simulink model "DAC_fxn_neg"  (R2018b)
settings: Solver=VariableStepAuto  StartTime=0.0  StopTime=10.0  RelTol=1e-3
libraries: simulink_extras x36, simulink x1
settings Model: Creator=iamcy  LastModifiedBy=iamcy

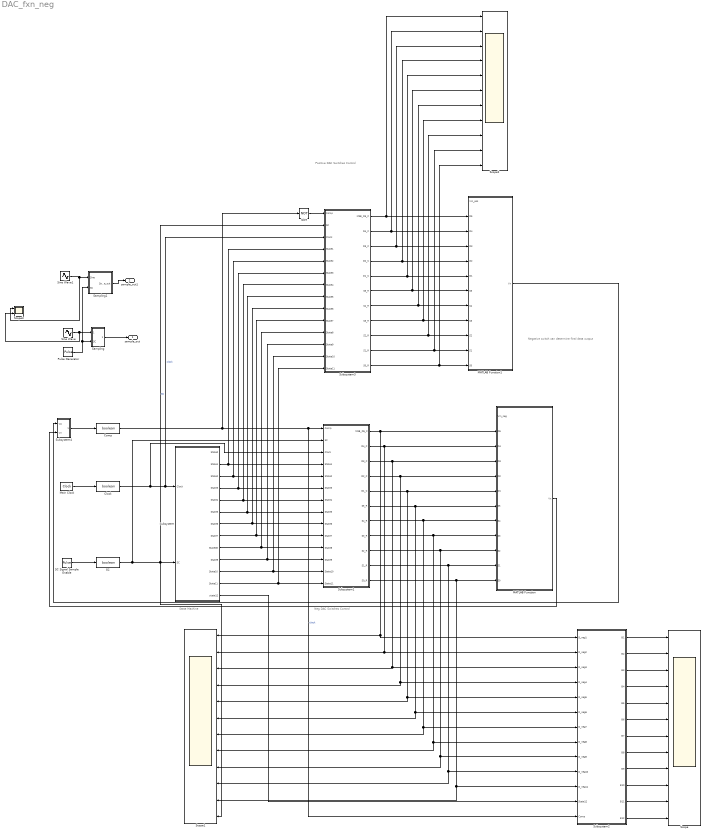
== system DAC_fxn_neg ==
  note: Negative switch can determine final data output
  note: Neg DAC Switches Control
  note: State Machine
  note: Positive DAC Switches Control
  Clock : DataTypeConversion  OutDataTypeStr=boolean
  Comp : DataTypeConversion  OutDataTypeStr=boolean
  MATLAB Function : MATLAB Function  TreatAsAtomicUnit=on
  MATLAB Function1 : MATLAB Function  TreatAsAtomicUnit=on
  Main Clock : simulink_extras/Flip Flops/Clock  period=1
  NOT : Logic  Operator=NOT  IconShape=distinctive  AllPortsSameDT=off  OutDataTypeStr=boolean
  Pulse Generator : DiscretePulseGenerator  PulseType=Time based  Period=13  PulseWidth=100/13
  SC : DataTypeConversion  OutDataTypeStr=boolean
  SC Signal Sample Enable : DiscretePulseGenerator  PulseType=Time based  Period=13  PulseWidth=100/13
  Sampling : Subsystem
  Sampling1 : Subsystem
  Scope : Scope  NumInputPorts=12
  Scope1 : Scope  NumInputPorts=12
  Scope2 : Scope  NumInputPorts=11
  Scope3 : Scope  NumInputPorts=2
  Sine Wave : Sin  Frequency=0.01  Phase=pi  SampleTime=0
  Sine Wave1 : Sin  Frequency=0.01  SampleTime=0
  Subsystem : Subsystem
  Subsystem1 : Subsystem
  Subsystem2 : Subsystem
  Subsystem3 : Subsystem
  Subsystem4 : Subsystem
  sample_out : Outport
  sample_out1 : Outport  Port=2
  wires:
  Subsystem/13(state12) -> Subsystem2/12(State12)
  Subsystem1/9(S2_R) -> MATLAB Function/10(S2), Scope1/9, Subsystem2/9(D_neg9)
  Subsystem1/11(S0_R) -> MATLAB Function/12(S0), Scope1/11, Subsystem2/11(D_neg11)
  Subsystem1/8(S3_R) -> MATLAB Function/9(S3), Scope1/8, Subsystem2/8(D_neg8)
  Subsystem1/6(S5_R) -> MATLAB Function/7(S5), Scope1/6, Subsystem2/6(D_neg6)
  Subsystem1/5(D1_C) -> MATLAB Function/6(D1), Scope1/5, Subsystem2/5(D_neg5)
  Subsystem1/3(D3_C) -> MATLAB Function/4(D3), Scope1/3, Subsystem2/3(D_neg3)
  Subsystem1/2(D4_C) -> MATLAB Function/3(D4), Scope1/2, Subsystem2/2(D_neg2)
  Subsystem1/1(MSB_D5_C) -> MATLAB Function/2(D5), Scope1/1, Subsystem2/1(D_neg1)
  Subsystem4/1(Comp) -> Comp/1
  Subsystem1/4(D2_C) -> MATLAB Function/5(D2), Scope1/4, Subsystem2/4(D_neg4)
  Comp/1 -> NOT/1, Subsystem2/13(Comp), Subsystem1/1(Comp)  "clock"
  Subsystem2/9(B9) -> Scope/9
  Subsystem2/12(B12) -> Scope/12
  Subsystem2/10(B10) -> Scope/10
  Subsystem2/7(B7) -> Scope/7
  Subsystem2/6(B6) -> Scope/6
  Subsystem2/3(B3) -> Scope/3
  Subsystem2/5(B5) -> Scope/5
  Subsystem2/2(B2) -> Scope/2
  Subsystem2/1(B1) -> Scope/1
  SC Signal Sample Enable/1 -> SC/1
  Main Clock/1 -> Clock/1
  Clock/1 -> Subsystem1/3(Clock), Subsystem3/3(Clock), Subsystem/1(Clock)  "clock"
  Subsystem2/4(B4) -> Scope/4
  Subsystem3/7(S4_R) -> MATLAB Function1/8(S4), Scope2/7
  Subsystem3/5(D1_C) -> MATLAB Function1/6(D1), Scope2/5
  Subsystem1/7(S4_R) -> MATLAB Function/8(S4), Scope1/7, Subsystem2/7(D_neg7)
  Subsystem3/9(S2_R) -> MATLAB Function1/10(S2), Scope2/9
  Subsystem2/11(B11) -> Scope/11
  Subsystem1/10(S1_R) -> MATLAB Function/11(S1), Scope1/10, Subsystem2/10(D_neg10)
  Subsystem3/3(D3_C) -> MATLAB Function1/4(D3), Scope2/3
  Subsystem3/1(MSB_D5_C) -> MATLAB Function1/2(D5), Scope2/1
  Subsystem2/8(B8) -> Scope/8
  NOT/1 -> Subsystem3/1(Comp)
  Subsystem3/8(S3_R) -> MATLAB Function1/9(S3), Scope2/8
  Subsystem3/6(S5_R) -> MATLAB Function1/7(S5), Scope2/6
  Subsystem3/10(S1_R) -> MATLAB Function1/11(S1), Scope2/10
  Subsystem3/2(D4_C) -> MATLAB Function1/3(D4), Scope2/2
  Subsystem3/4(D2_C) -> MATLAB Function1/5(D2), Scope2/4
  Subsystem3/11(S0_R) -> MATLAB Function1/12(S0), Scope2/11
  Subsystem/11(State10) -> Subsystem3/13(State10), Subsystem1/13(State10)
  Subsystem/9(State08) -> Subsystem3/11(State8), Subsystem1/11(State8)
  Subsystem/10(State9) -> Subsystem3/12(State9), Subsystem1/12(State9)
  Subsystem/7(State6) -> Subsystem3/9(State6), Subsystem1/9(State6)
  Subsystem/12(State11) -> Subsystem3/14(State11), Subsystem1/14(State11)
  Subsystem/8(State7) -> Subsystem3/10(State7), Subsystem1/10(State7)
  Subsystem/4(State3) -> Subsystem3/6(State3), Subsystem1/6(State3)
  Subsystem/5(State4) -> Subsystem3/7(State4), Subsystem1/7(State4)
  SC/1 -> Subsystem1/2(SC), Scope1/12, Subsystem3/2(SC), Subsystem/2(SC)  "SC"
  Subsystem/3(State2) -> Subsystem3/5(State2), Subsystem1/5(State2)
  Subsystem/6(State5) -> Subsystem3/8(State5), Subsystem1/8(State5)
  Subsystem/2(State1) -> Subsystem3/4(State1), Subsystem1/4(State1)
  MATLAB Function1/1(Vx) -> Subsystem4/1(Vp)
  MATLAB Function/1(Vx) -> Subsystem4/2(Vn)
  Sampling/1(Sample_out) -> sample_out/1
  Sine Wave/1 -> Scope3/2, Sampling/1(Sine)
  Pulse Generator/1 -> Sampling1/2(SC), Sampling/2(SC)
  Sampling1/1(Sample_out) -> sample_out1/1
  Sine Wave1/1 -> Scope3/1, Sampling1/1(Sine)

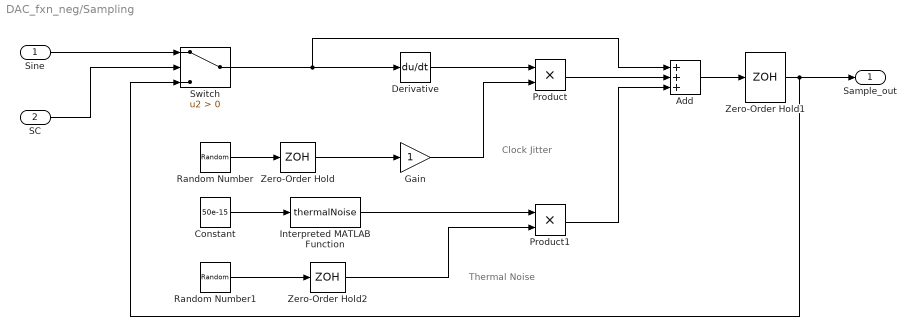
== system DAC_fxn_neg/Sampling ==
  note: Clock Jitter
  note: Thermal Noise
  Sine : Inport
  SC : Inport  Port=2
  Add : Sum  Inputs=3
  Constant : Constant  Value=50e-15
  Derivative : Derivative  CoefficientInTFapproximation=0
  Gain : Gain
  Interpreted MATLAB Function : MATLABFcn  MATLABFcn=thermalNoise
  Product : Product
  Product1 : Product
  Random Number : RandomNumber  Variance=30e-12  SampleTime=0.1
  Random Number1 : RandomNumber  Variance=30e-12  SampleTime=0.1
  Switch : Switch  Criteria=u2 > Threshold
  Zero-Order Hold : ZeroOrderHold  SampleTime=-1
  Zero-Order Hold1 : ZeroOrderHold  SampleTime=13
  Zero-Order Hold2 : ZeroOrderHold  SampleTime=-1
  Sample_out : Outport
  wires:
  Random Number/1 -> Zero-Order Hold/1
  Random Number1/1 -> Zero-Order Hold2/1
  Zero-Order Hold2/1 -> Product1/2
  Derivative/1 -> Product/1
  Interpreted MATLAB Function/1 -> Product1/1
  Product/1 -> Add/2
  Constant/1 -> Interpreted MATLAB Function/1
  Zero-Order Hold1/1 -> Sample_out/1, Switch/3
  Switch/1 -> Add/1, Derivative/1
  Zero-Order Hold/1 -> Gain/1
  Add/1 -> Zero-Order Hold1/1
  Gain/1 -> Product/2
  Product1/1 -> Add/3
  SC/1 -> Switch/2
  Sine/1 -> Switch/1

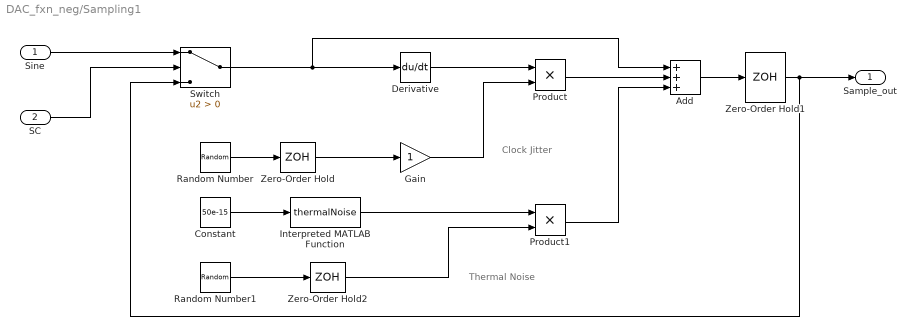
== system DAC_fxn_neg/Sampling1 ==
  note: Clock Jitter
  note: Thermal Noise
  Sine : Inport
  SC : Inport  Port=2
  Add : Sum  Inputs=3
  Constant : Constant  Value=50e-15
  Derivative : Derivative  CoefficientInTFapproximation=0
  Gain : Gain
  Interpreted MATLAB Function : MATLABFcn  MATLABFcn=thermalNoise
  Product : Product
  Product1 : Product
  Random Number : RandomNumber  Variance=30e-12  SampleTime=0.1
  Random Number1 : RandomNumber  Variance=30e-12  SampleTime=0.1
  Switch : Switch  Criteria=u2 > Threshold
  Zero-Order Hold : ZeroOrderHold  SampleTime=-1
  Zero-Order Hold1 : ZeroOrderHold  SampleTime=13
  Zero-Order Hold2 : ZeroOrderHold  SampleTime=-1
  Sample_out : Outport
  wires:
  Random Number/1 -> Zero-Order Hold/1
  Random Number1/1 -> Zero-Order Hold2/1
  Zero-Order Hold2/1 -> Product1/2
  Derivative/1 -> Product/1
  Interpreted MATLAB Function/1 -> Product1/1
  Product/1 -> Add/2
  Constant/1 -> Interpreted MATLAB Function/1
  Zero-Order Hold1/1 -> Sample_out/1, Switch/3
  Switch/1 -> Add/1, Derivative/1
  Zero-Order Hold/1 -> Gain/1
  Add/1 -> Zero-Order Hold1/1
  Gain/1 -> Product/2
  Product1/1 -> Add/3
  SC/1 -> Switch/2
  Sine/1 -> Switch/1

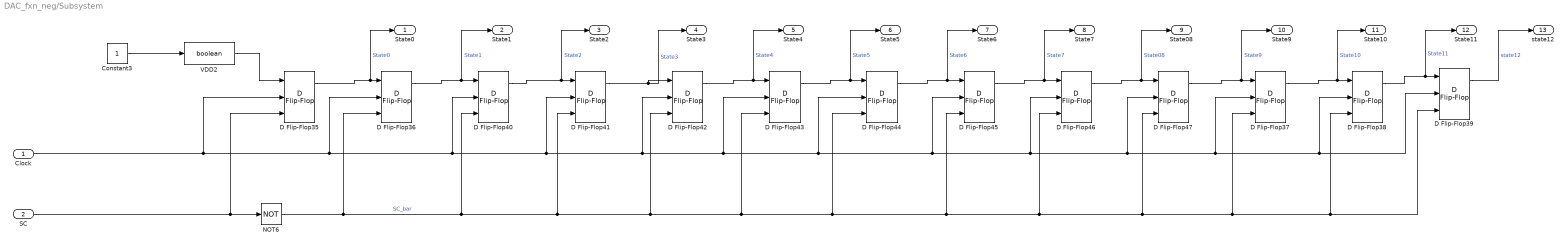
== system DAC_fxn_neg/Subsystem ==
  Clock : Inport
  SC : Inport  Port=2
  Constant3 : Constant
  D Flip-Flop{35..47} (13 alike) : simulink_extras/Flip Flops/D Flip-Flop
      settings: SourceProductName=Simulink
  NOT6 : Logic  Operator=NOT  IconShape=distinctive  AllPortsSameDT=off  OutDataTypeStr=boolean
  VDD2 : DataTypeConversion  OutDataTypeStr=boolean
  State0 : Outport
  State1 : Outport  Port=2
  State2 : Outport  Port=3
  State3 : Outport  Port=4
  State4 : Outport  Port=5
  State5 : Outport  Port=6
  State6 : Outport  Port=7
  State7 : Outport  Port=8
  State08 : Outport  Port=9
  State9 : Outport  Port=10
  State10 : Outport  Port=11
  State11 : Outport  Port=12
  state12 : Outport  Port=13
  wires:
  D Flip-Flop43/1 -> State5/1, D Flip-Flop44/1  "State5"
  D Flip-Flop40/1 -> State2/1, D Flip-Flop41/1  "State2"
  D Flip-Flop45/1 -> State7/1, D Flip-Flop46/1  "State7"
  D Flip-Flop38/1 -> State11/1, D Flip-Flop39/1  "State11"
  D Flip-Flop42/1 -> State4/1, D Flip-Flop43/1  "State4"
  D Flip-Flop44/1 -> State6/1, D Flip-Flop45/1  "State6"
  NOT6/1 -> D Flip-Flop42/3, D Flip-Flop44/3, D Flip-Flop46/3, D Flip-Flop38/3, D Flip-Flop39/3, D Flip-Flop37/3, D Flip-Flop47/3, D Flip-Flop45/3, D Flip-Flop43/3, D Flip-Flop41/3, D Flip-Flop40/3, D Flip-Flop36/3  "SC_bar"
  D Flip-Flop36/1 -> State1/1, D Flip-Flop40/1  "State1"
  Clock/1 -> D Flip-Flop36/2, D Flip-Flop41/2, D Flip-Flop42/2, D Flip-Flop43/2, D Flip-Flop44/2, D Flip-Flop45/2, D Flip-Flop46/2, D Flip-Flop38/2, D Flip-Flop39/2, D Flip-Flop37/2, D Flip-Flop47/2, D Flip-Flop40/2, D Flip-Flop35/2
  D Flip-Flop47/1 -> State9/1, D Flip-Flop37/1  "State9"
  Constant3/1 -> VDD2/1
  D Flip-Flop41/1 -> State3/1, D Flip-Flop42/1  "State3"
  D Flip-Flop37/1 -> State10/1, D Flip-Flop38/1  "State10"
  D Flip-Flop35/1 -> State0/1, D Flip-Flop36/1  "State0"
  D Flip-Flop46/1 -> State08/1, D Flip-Flop47/1  "State08"
  SC/1 -> NOT6/1, D Flip-Flop35/3
  VDD2/1 -> D Flip-Flop35/1
  D Flip-Flop39/1 -> state12/1  "state12"

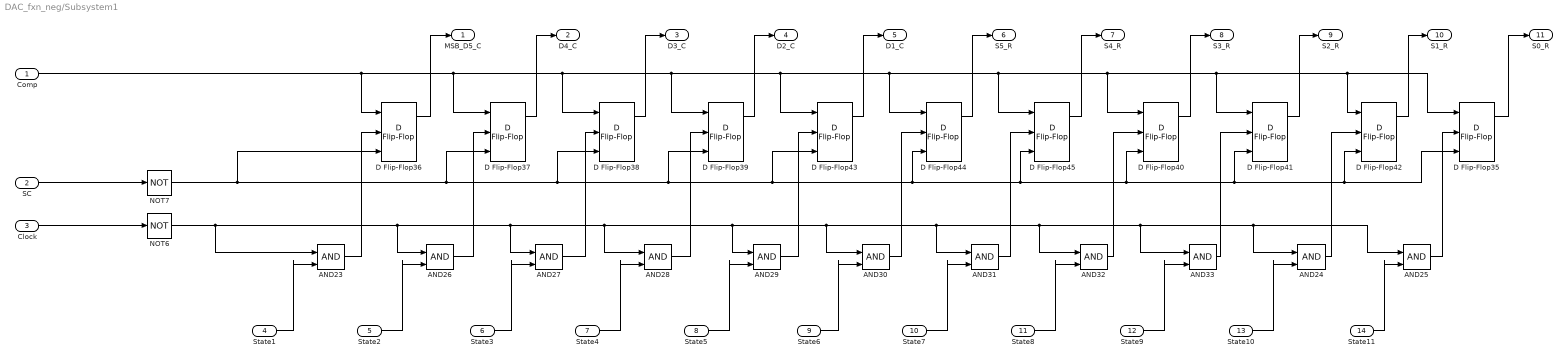
== system DAC_fxn_neg/Subsystem1 ==
  Comp : Inport
  SC : Inport  Port=2
  Clock : Inport  Port=3
  State1 : Inport  Port=4
  State2 : Inport  Port=5
  State3 : Inport  Port=6
  State4 : Inport  Port=7
  State5 : Inport  Port=8
  State6 : Inport  Port=9
  State7 : Inport  Port=10
  State8 : Inport  Port=11
  State9 : Inport  Port=12
  State10 : Inport  Port=13
  State11 : Inport  Port=14
  AND{23..33} (11 alike) : Logic  IconShape=distinctive  AllPortsSameDT=off  OutDataTypeStr=boolean
  D Flip-Flop{35..45} (11 alike) : simulink_extras/Flip Flops/D Flip-Flop
      settings: SourceProductName=Simulink
  NOT6 : Logic  Operator=NOT  IconShape=distinctive  AllPortsSameDT=off  OutDataTypeStr=boolean
  NOT7 : Logic  Operator=NOT  IconShape=distinctive  AllPortsSameDT=off  OutDataTypeStr=boolean
  MSB_D5_C : Outport
  D4_C : Outport  Port=2
  D3_C : Outport  Port=3
  D2_C : Outport  Port=4
  D1_C : Outport  Port=5
  S5_R : Outport  Port=6
  S4_R : Outport  Port=7
  S3_R : Outport  Port=8
  S2_R : Outport  Port=9
  S1_R : Outport  Port=10
  S0_R : Outport  Port=11
  wires:
  NOT7/1 -> D Flip-Flop35/3, D Flip-Flop42/3, D Flip-Flop41/3, D Flip-Flop40/3, D Flip-Flop45/3, D Flip-Flop44/3, D Flip-Flop43/3, D Flip-Flop39/3, D Flip-Flop38/3, D Flip-Flop37/3, D Flip-Flop36/3
  D Flip-Flop41/1 -> S2_R/1
  AND23/1 -> D Flip-Flop36/2
  State9/1 -> AND33/2
  Comp/1 -> D Flip-Flop35/1, D Flip-Flop42/1, D Flip-Flop41/1, D Flip-Flop40/1, D Flip-Flop45/1, D Flip-Flop44/1, D Flip-Flop43/1, D Flip-Flop39/1, D Flip-Flop38/1, D Flip-Flop37/1, D Flip-Flop36/1
  D Flip-Flop42/1 -> S1_R/1
  AND27/1 -> D Flip-Flop38/2
  NOT6/1 -> AND25/1, AND24/1, AND33/1, AND32/1, AND31/1, AND30/1, AND29/1, AND28/1, AND27/1, AND26/1, AND23/1
  AND25/1 -> D Flip-Flop35/2
  AND29/1 -> D Flip-Flop43/2
  AND31/1 -> D Flip-Flop45/2
  AND28/1 -> D Flip-Flop39/2
  State1/1 -> AND23/2
  AND33/1 -> D Flip-Flop41/2
  D Flip-Flop45/1 -> S4_R/1
  State5/1 -> AND29/2
  AND26/1 -> D Flip-Flop37/2
  AND24/1 -> D Flip-Flop42/2
  SC/1 -> NOT7/1
  AND32/1 -> D Flip-Flop40/2
  State10/1 -> AND24/2
  AND30/1 -> D Flip-Flop44/2
  D Flip-Flop38/1 -> D3_C/1
  Clock/1 -> NOT6/1
  D Flip-Flop36/1 -> MSB_D5_C/1
  D Flip-Flop37/1 -> D4_C/1
  D Flip-Flop35/1 -> S0_R/1
  D Flip-Flop43/1 -> D1_C/1
  State4/1 -> AND28/2
  State3/1 -> AND27/2
  State2/1 -> AND26/2
  State8/1 -> AND32/2
  D Flip-Flop44/1 -> S5_R/1
  State6/1 -> AND30/2
  State11/1 -> AND25/2
  D Flip-Flop40/1 -> S3_R/1
  State7/1 -> AND31/2
  D Flip-Flop39/1 -> D2_C/1

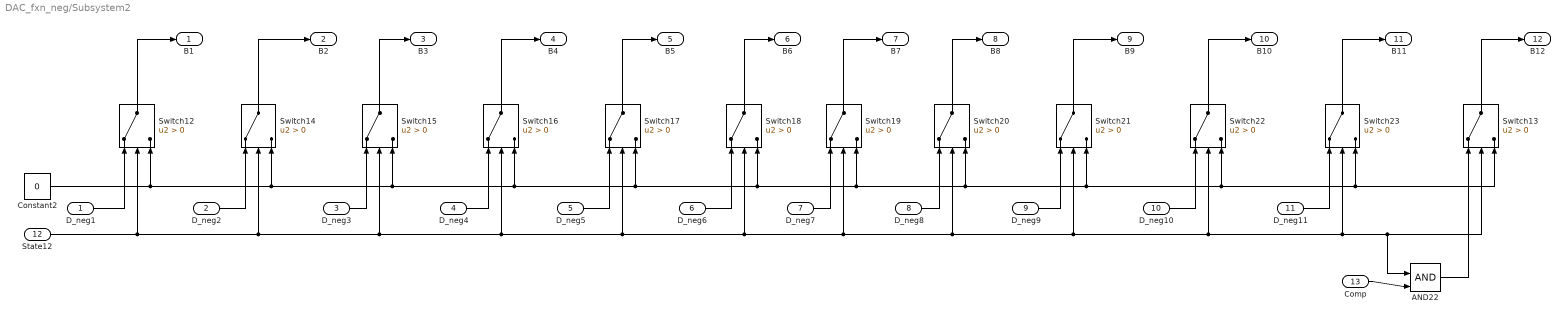
== system DAC_fxn_neg/Subsystem2 ==
  D_neg1 : Inport
  D_neg2 : Inport  Port=2
  D_neg3 : Inport  Port=3
  D_neg4 : Inport  Port=4
  D_neg5 : Inport  Port=5
  D_neg6 : Inport  Port=6
  D_neg7 : Inport  Port=7
  D_neg8 : Inport  Port=8
  D_neg9 : Inport  Port=9
  D_neg10 : Inport  Port=10
  D_neg11 : Inport  Port=11
  State12 : Inport  Port=12
  Comp : Inport  Port=13
  AND22 : Logic  IconShape=distinctive  AllPortsSameDT=off  OutDataTypeStr=boolean
  Constant2 : Constant  Value=0
  Switch{12..23} (12 alike) : Switch  Criteria=u2 > Threshold
  B1 : Outport
  B2 : Outport  Port=2
  B3 : Outport  Port=3
  B4 : Outport  Port=4
  B5 : Outport  Port=5
  B6 : Outport  Port=6
  B7 : Outport  Port=7
  B8 : Outport  Port=8
  B9 : Outport  Port=9
  B10 : Outport  Port=10
  B11 : Outport  Port=11
  B12 : Outport  Port=12
  wires:
  Constant2/1 -> Switch12/3, Switch13/3, Switch23/3, Switch22/3, Switch21/3, Switch20/3, Switch19/3, Switch18/3, Switch17/3, Switch16/3, Switch15/3, Switch14/3
  Switch22/1 -> B10/1
  Switch17/1 -> B5/1
  Switch12/1 -> B1/1
  Switch14/1 -> B2/1
  Switch18/1 -> B6/1
  Switch16/1 -> B4/1
  Switch15/1 -> B3/1
  Switch23/1 -> B11/1
  Switch20/1 -> B8/1
  Switch21/1 -> B9/1
  Switch19/1 -> B7/1
  Switch13/1 -> B12/1
  State12/1 -> Switch12/2, Switch14/2, Switch15/2, Switch16/2, Switch17/2, Switch19/2, Switch20/2, Switch21/2, Switch22/2, AND22/1, Switch13/2, Switch23/2, Switch18/2
  AND22/1 -> Switch13/1
  Comp/1 -> AND22/2
  D_neg11/1 -> Switch23/1
  D_neg10/1 -> Switch22/1
  D_neg9/1 -> Switch21/1
  D_neg8/1 -> Switch20/1
  D_neg7/1 -> Switch19/1
  D_neg6/1 -> Switch18/1
  D_neg5/1 -> Switch17/1
  D_neg4/1 -> Switch16/1
  D_neg3/1 -> Switch15/1
  D_neg2/1 -> Switch14/1
  D_neg1/1 -> Switch12/1

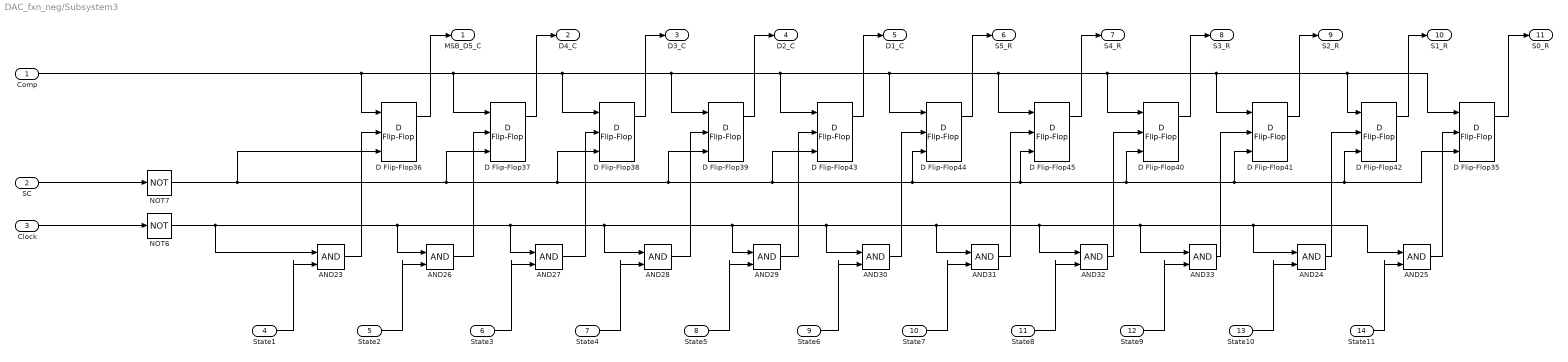
== system DAC_fxn_neg/Subsystem3 ==
  Comp : Inport
  SC : Inport  Port=2
  Clock : Inport  Port=3
  State1 : Inport  Port=4
  State2 : Inport  Port=5
  State3 : Inport  Port=6
  State4 : Inport  Port=7
  State5 : Inport  Port=8
  State6 : Inport  Port=9
  State7 : Inport  Port=10
  State8 : Inport  Port=11
  State9 : Inport  Port=12
  State10 : Inport  Port=13
  State11 : Inport  Port=14
  AND{23..33} (11 alike) : Logic  IconShape=distinctive  AllPortsSameDT=off  OutDataTypeStr=boolean
  D Flip-Flop{35..45} (11 alike) : simulink_extras/Flip Flops/D Flip-Flop
      settings: SourceProductName=Simulink
  NOT6 : Logic  Operator=NOT  IconShape=distinctive  AllPortsSameDT=off  OutDataTypeStr=boolean
  NOT7 : Logic  Operator=NOT  IconShape=distinctive  AllPortsSameDT=off  OutDataTypeStr=boolean
  MSB_D5_C : Outport
  D4_C : Outport  Port=2
  D3_C : Outport  Port=3
  D2_C : Outport  Port=4
  D1_C : Outport  Port=5
  S5_R : Outport  Port=6
  S4_R : Outport  Port=7
  S3_R : Outport  Port=8
  S2_R : Outport  Port=9
  S1_R : Outport  Port=10
  S0_R : Outport  Port=11
  wires:
  NOT7/1 -> D Flip-Flop35/3, D Flip-Flop42/3, D Flip-Flop41/3, D Flip-Flop40/3, D Flip-Flop45/3, D Flip-Flop44/3, D Flip-Flop43/3, D Flip-Flop39/3, D Flip-Flop38/3, D Flip-Flop37/3, D Flip-Flop36/3
  D Flip-Flop41/1 -> S2_R/1
  AND23/1 -> D Flip-Flop36/2
  State9/1 -> AND33/2
  Comp/1 -> D Flip-Flop35/1, D Flip-Flop42/1, D Flip-Flop41/1, D Flip-Flop40/1, D Flip-Flop45/1, D Flip-Flop44/1, D Flip-Flop43/1, D Flip-Flop39/1, D Flip-Flop38/1, D Flip-Flop37/1, D Flip-Flop36/1
  D Flip-Flop42/1 -> S1_R/1
  AND27/1 -> D Flip-Flop38/2
  NOT6/1 -> AND25/1, AND24/1, AND33/1, AND32/1, AND31/1, AND30/1, AND29/1, AND28/1, AND27/1, AND26/1, AND23/1
  AND25/1 -> D Flip-Flop35/2
  AND29/1 -> D Flip-Flop43/2
  AND31/1 -> D Flip-Flop45/2
  AND28/1 -> D Flip-Flop39/2
  State1/1 -> AND23/2
  AND33/1 -> D Flip-Flop41/2
  D Flip-Flop45/1 -> S4_R/1
  State5/1 -> AND29/2
  AND26/1 -> D Flip-Flop37/2
  AND24/1 -> D Flip-Flop42/2
  SC/1 -> NOT7/1
  AND32/1 -> D Flip-Flop40/2
  State10/1 -> AND24/2
  AND30/1 -> D Flip-Flop44/2
  D Flip-Flop38/1 -> D3_C/1
  Clock/1 -> NOT6/1
  D Flip-Flop36/1 -> MSB_D5_C/1
  D Flip-Flop37/1 -> D4_C/1
  D Flip-Flop35/1 -> S0_R/1
  D Flip-Flop43/1 -> D1_C/1
  State4/1 -> AND28/2
  State3/1 -> AND27/2
  State2/1 -> AND26/2
  State8/1 -> AND32/2
  D Flip-Flop44/1 -> S5_R/1
  State6/1 -> AND30/2
  State11/1 -> AND25/2
  D Flip-Flop40/1 -> S3_R/1
  State7/1 -> AND31/2
  D Flip-Flop39/1 -> D2_C/1

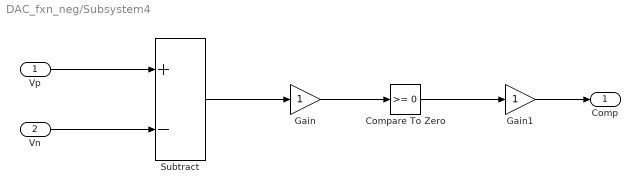
== system DAC_fxn_neg/Subsystem4 ==
  Vp : Inport
  Vn : Inport  Port=2
  Compare To Zero : simulink/Logic and Bit Operations/Compare To Zero  relop=>=  OutDataTypeStr=boolean
  Gain : Gain
  Gain1 : Gain
  Subtract : Sum  Inputs=+-
  Comp : Outport
  wires:
  Gain1/1 -> Comp/1
  Subtract/1 -> Gain/1
  Gain/1 -> Compare To Zero/1
  Compare To Zero/1 -> Gain1/1
  Vn/1 -> Subtract/2
  Vp/1 -> Subtract/1

== matlab function DAC_fxn_neg/MATLAB Function1 ==
  data: Vin_pos input; Vx output; D5 input; D4 input; D3 input; D2 input; D1 input; S5 input; S4 input; S3 input; S2 input; S1 input; S0 input
function Vx  = DAC_pos_function(Vin_pos,D5,D4,D3,D2,D1,S5,S4,S3,S2,S1,S0)
%%%%%%%%%%%%%%%%%%%%%%%%%%%%%%%%%%%%%%%%%%%%%%%%%%%%%%
% 2018/12/3
% Purpose:  This file is to module R C DAC
%          
%   Copyright (c) 2018 by Shanshan Xie
%   for SAR ADC project in ADC course
%%%%%%%%%%%%%%%%%%%%%%%%%%%%%%%%%%%%%%%%%%%%%%%%%%%%%%

clear;

sigma_C = 0.001322917989585;
sigma_R = 0.001841423909340;

N_CDAC = 5;
N_RDAC = 6;
N_DAC = N_CDAC+N_RDAC;

Cu = 57.596e-15;
Ru = 200;

Vref = 1;
% Vin_pos = 1;

%% Switch for C DAC
%  D5 D4 D3 D2 D1
D = [D5 D4 D3 D2 D1]; 

%% Switch for R DAC
% thisSwitch = 1; %swich from 0 to 3 Vref0  = 0, Vref63 = 63/64Vref

%Switch Decoder
thisSwitch = S5*2^5 + S4*2^4 + S3*2^3 + S2*2^2 + S1*2^1 + S0*2^0;

% S = [zeros(1,63),1];
% for i=2:64
%     S(i,:) = [S(i-1, 2:64),0];
% end

%% Generate C, R with mismatch 32 number of C and 64 number of R
C = normrnd(1,sigma_C,[1,(2^N_CDAC)]);
% C = normrnd(1,sigma_C,[1,(2^N_CDAC)]);

R = normrnd(1,sigma_R,[1,(2^N_RDAC)]);
% R = normrnd(1,sigma_R,[1,(2^N_RDAC)]);


C_binary = C(1);
N_b = 2;

%% generate binary Cap value for cap DAC
for i = 1:N_CDAC-1
    C_binary = [sum(C(N_b:(N_b+N_b-1))), C_binary];
    N_b = N_b*2;
    i=i+1;
end
C0 = C(2^N_CDAC);
Ctotal = sum(C);

%% Generate Thermometer R DAC
i = 1;
while i<length(R)
   R_seq(:,i) = [sum(R(1:i))];
   i = i+1;
end
R_seq = [0, R_seq];
% R_seq = fliplr(R_seq);
% R_seq = repmat(R_seq(1:2^N_RDAC),2^N_RDAC,1);

Rtotal = sum(R);

%% Generate Cap voltage
for i = 1:5
   CD(:,i) = C_binary(i)*D(i);
   i = i+1;
end

Vx_cap = (sum(CD)*Vref) / Ctotal;

%% Generate Resistor Voltage
Vx_res = (Vref * C0 * R_seq(thisSwitch+1)) / (Rtotal * Ctotal);

Vx = Vx_cap + Vx_res + Vin_pos;


end

== matlab function DAC_fxn_neg/MATLAB Function ==
  data: Vin_neg input; Vx output; D5 input; D4 input; D3 input; D2 input; D1 input; S5 input; S4 input; S3 input; S2 input; S1 input; S0 input
function Vx  = DAC_neg_function(Vin_neg,D5,D4,D3,D2,D1,S5,S4,S3,S2,S1,S0)
%%%%%%%%%%%%%%%%%%%%%%%%%%%%%%%%%%%%%%%%%%%%%%%%%%%%%%
% 2018/12/3
% Purpose:  This file is to module R C DAC
%          
%   Copyright (c) 2018 by Shanshan Xie
%   for SAR ADC project in ADC course
%%%%%%%%%%%%%%%%%%%%%%%%%%%%%%%%%%%%%%%%%%%%%%%%%%%%%%

clear;

sigma_C = 0.001322917989585;
sigma_R = 0.001841423909340;

N_CDAC = 5;
N_RDAC = 6;
N_DAC = N_CDAC+N_RDAC;

Cu = 57.596e-15;
Ru = 200;

Vref = 1;
% Vin_neg = 1;

%% Switch for C DAC
%  D5 D4 D3 D2 D1
D = [D5 D4 D3 D2 D1]; 

%% Switch for R DAC
% thisSwitch = 1; %swich from 0 to 3 Vref0  = 0, Vref63 = 63/64Vref
thisSwitch = S5*2^5 + S4*2^4 + S3*2^3 + S2*2^2 + S1*2^1 + S0*2^0;

% S = [zeros(1,63),1];
% for i=2:64
%     S(i,:) = [S(i-1, 2:64),0];
% end

%% Generate C, R with mismatch 32 number of C and 64 number of R
C = normrnd(1,sigma_C,[1,(2^N_CDAC)]);
% C = normrnd(1,sigma_C,[1,(2^N_CDAC)]);

R = normrnd(1,sigma_R,[1,(2^N_RDAC)]);
% R = normrnd(1,sigma_R,[1,(2^N_RDAC)]);


C_binary = C(1);
N_b = 2;

%% generate binary Cap value for cap DAC
for i = 1:N_CDAC-1
    C_binary = [sum(C(N_b:(N_b+N_b-1))), C_binary];
    N_b = N_b*2;
    i=i+1;
end
C0 = C(2^N_CDAC);
Ctotal = sum(C);

%% Generate Thermometer R DAC
i = 1;
while i<length(R)
   R_seq(:,i) = [sum(R(1:i))];
   i = i+1;
end
R_seq = [0, R_seq];
% R_seq = fliplr(R_seq);
% R_seq = repmat(R_seq(1:2^N_RDAC),2^N_RDAC,1);

Rtotal = sum(R);

%% Generate Cap voltage
for i = 1:5
   CD(:,i) = C_binary(i)*D(i);
   i = i+1;
end

Vx_cap = (sum(CD)*Vref) / Ctotal;

%% Generate Resistor Voltage
Vx_res = (Vref * C0 * R_seq(thisSwitch+1)) / (Rtotal * Ctotal);

Vx = Vx_cap + Vx_res + Vin_neg;


end
